simulink model "HeaterPOMTM"  (R2014a)
settings: Solver=ode45  StartTime=0.0  StopTime=ttotal  RelTol=1e-3
values from neighbouring files (symbols this model uses):
  K = Kpp    (= 0.76675)    [Modeling.m]    (also in model.m = 126)
  ks = 1    [Modeling.m]    (also in model.m)
  T0 = 3.865    [model.m]
  ttotal = 200    [Modeling.m]    (also in model.m)
undefined symbols (not defined in the file or in its folder): TAU
settings Model: Creator=jEdwin  LastModifiedBy=jEdwin

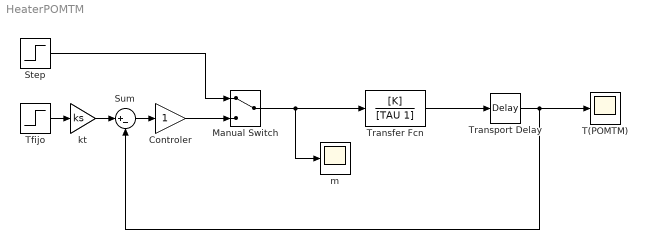
== system HeaterPOMTM ==
  Controler : Gain
  Manual Switch : ManualSwitch
  Step : Step  Time=ttotal/3  After=2  SampleTime=0
  Sum : Sum  Inputs=|+-  SaturateOnIntegerOverflow=on
  T(POMTM) : Scope
      settings: TimeRange=60  YMin=0  YMax=700  SaveName=Tm1
  Tfijo : Step  Time=0  After=5  SampleTime=0
  Transfer Fcn : TransferFcn  Numerator=[K]  Denominator=[TAU 1]
  Transport Delay : TransportDelay  DelayTime=T0
  kt : Gain  Gain=ks  SaturateOnIntegerOverflow=on  OutDataTypeStr=Inherit: Same as input  ParamDataTypeStr=Inherit: Same as input
  m : Scope
      settings: SaveName=m
  wires:
  Controler/1 -> Manual Switch/2
  Manual Switch/1 -> Transfer Fcn/1, m/1
  Sum/1 -> Controler/1
  Transport Delay/1 -> Sum/2, T(POMTM)/1
  Step/1 -> Manual Switch/1
  Tfijo/1 -> kt/1
  kt/1 -> Sum/1
  Transfer Fcn/1 -> Transport Delay/1
